simulink model "test"  (Simulink 10.1)
settings: Solver=FixedStepAuto  StartTime=0.0  StopTime=Config.simulationTime  FixedStep=Config.tStep  RelTol=1e-3
InitFcn:
  | init
undefined symbols (not defined in the file or in its folder): Config, confVisualizer, DiscIntNeverNeededParam
libraries: WBToolboxLibrary x12
settings Model: Creator=giuseppe  LastModifiedBy=giuseppe
settings DataIOCC: SaveFormat=Dataset  ReturnWorkspaceOutputs=on
settings OptimizationCC: LifeSpan=auto
settings DebuggingCC: UnderspecifiedInitializationDetection=Simplified  MergeDetectMultiDrivingBlocksExec=error  SFUnexpectedBacktrackingDiag=error  SFNoUnconditionalDefaultTransitionDiag=error  SFExecutionAtInitializationDiag=warning  ArithmeticOperatorsInVariantConditions=error
settings HardwareCC: ProdBitPerPointer=64  ProdBitPerSizeT=64  ProdBitPerPtrDiffT=64  ProdLargestAtomicFloat=Float  ProdIntDivRoundTo=Zero  ProdEndianess=LittleEndian  ProdWordSize=64  ProdHWDeviceType=Intel->x86-64 (Windows64)
settings ModelReferenceCC: PropagateSignalLabelsOutOfModel=on
settings SFSimCC: SimUseLocalCustomCode=on  CustomCodeUndefinedFunction=FilterOut
settings RTWCC: RTWUseLocalCustomCode=on
settings CodeAppCC: StateflowObjectComments=off
settings GRTTargetCC: TargetLangStandard=C99 (ISO)  CombineOutputUpdateFcns=on  GRTInterface=off
settings ConfigComp: CovMetricSettings=dwe  CovHtmlReporting=off  CovSaveCumulativeToWorkspaceVar=off  CovSaveSingleToWorkspaceVar=off  CovExternalEMLEnable=on

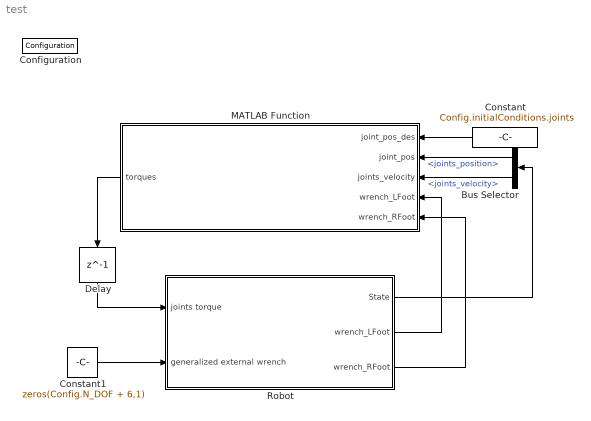
== system test ==
  Bus Selector : BusSelector  OutputSignals=joints_position,joints_velocity
  Configuration : WBToolboxLibrary/Utilities/Configuration  ConfigSource=Workspace  ConfigObject='WBTConfigRobot'
      settings: SourceProductName=WholeBodyToolbox
  Constant : Constant  Value=Config.initialConditions.joints
  Constant1 : Constant  Value=zeros(Config.N_DOF + 6,1)
  Delay : Delay  DelayLength=1  InitialCondition=zeros(23,1)
  MATLAB Function : MATLAB Function  TreatAsAtomicUnit=on
  Robot : Subsystem
  wires:
  Constant1/1 -> Robot/2(generalized external wrench)
  Bus Selector/1 -> MATLAB Function/2(joint_pos)  "<joints_position>"
  Bus Selector/2 -> MATLAB Function/3(joints_velocity)  "<joints_velocity>"
  Robot/1(State) -> Bus Selector/1
  Robot/2(wrench_LFoot) -> MATLAB Function/4(wrench_LFoot)
  Robot/3(wrench_RFoot) -> MATLAB Function/5(wrench_RFoot)
  Constant/1 -> MATLAB Function/1(joint_pos_des)
  MATLAB Function/1(torques) -> Delay/1
  Delay/1 -> Robot/1(joints torque)

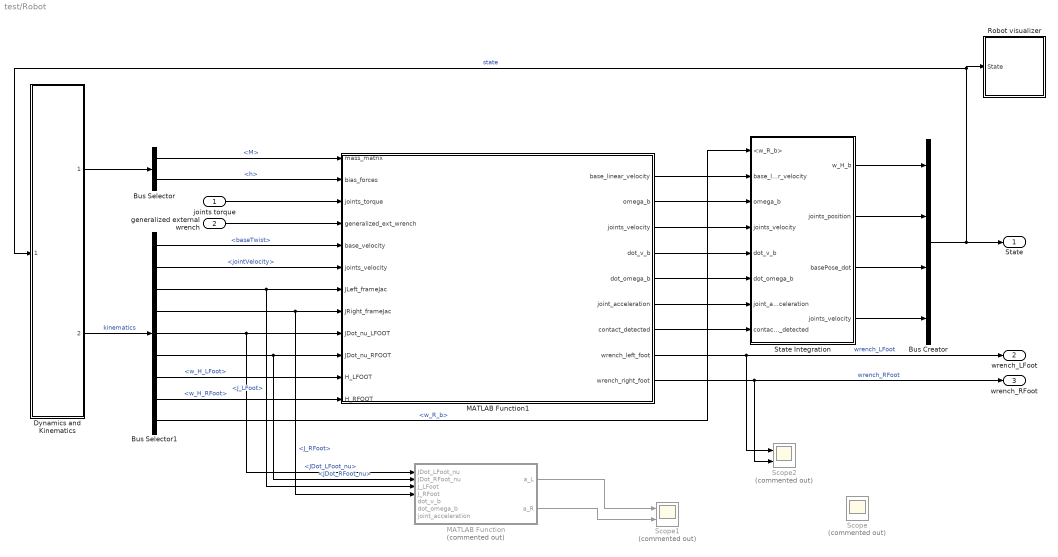
== system test/Robot ==
  joints torque : Inport
  generalized external wrench : Inport  Port=2
  Bus Creator : BusCreator  Inputs=4
  Bus Selector : BusSelector  OutputSignals=M,h
  Bus Selector1 : BusSelector  OutputSignals=baseTwist,jointVelocity,J_LFoot,J_RFoot,JDot_LFoot_nu,JDot_RFoot_nu,w_H_LFoot,w_H_RFoot,w_R_b
  Dynamics and Kinematics : Subsystem
  MATLAB Function : MATLAB Function  Commented=on  TreatAsAtomicUnit=on
  MATLAB Function1 : MATLAB Function  TreatAsAtomicUnit=on
  Robot visualizer : Subsystem  SystemSampleTime=confVisualizer.tStep
  Scope : Scope  Commented=on
  Scope1 : Scope  Commented=on  NumInputPorts=2
  Scope2 : Scope  Commented=on  NumInputPorts=2
  State Integration : Subsystem
  State : Outport
  wrench_LFoot : Outport  Port=2
  wrench_RFoot : Outport  Port=3
  wires:
  Bus Selector1/9 -> State Integration/1(<w_R_b>)  "<w_R_b>"
  State Integration/1(w_H_b) -> Bus Creator/1
  Bus Selector1/6 -> MATLAB Function/2(JDot_RFoot_nu), MATLAB Function1/10(JDot_nu_RFOOT)  "<JDot_RFoot_nu>"
  Bus Selector1/5 -> MATLAB Function/1(JDot_LFoot_nu), MATLAB Function1/9(JDot_nu_LFOOT)  "<JDot_LFoot_nu>"
  MATLAB Function1/8(wrench_left_foot) -> wrench_LFoot/1, Scope2/1  "wrench_LFoot"
  MATLAB Function1/9(wrench_right_foot) -> wrench_RFoot/1, Scope2/2  "wrench_RFoot"
  Bus Selector/1 -> MATLAB Function1/1(mass_matrix)  "<M>"
  Bus Selector/2 -> MATLAB Function1/2(bias_forces)  "<h>"
  Bus Selector1/4 -> MATLAB Function/4(J_RFoot), MATLAB Function1/8(JRight_frameJac)  "<J_RFoot>"
  Bus Creator/1 -> Robot visualizer/1(State), Dynamics and Kinematics/1(systemState), State/1  "state"
  State Integration/4("joints_velocity ") -> Bus Creator/4
  State Integration/2(joints_position) -> Bus Creator/2
  Bus Selector1/2 -> MATLAB Function1/6("joints_velocity ")  "<jointVelocity>"
  State Integration/3(basePose_dot) -> Bus Creator/3
  Bus Selector1/8 -> MATLAB Function1/12(H_RFOOT)  "<w_H_RFoot>"
  Dynamics and Kinematics/2(kinematics) -> Bus Selector1/1  "kinematics"
  generalized external wrench/1 -> MATLAB Function1/4(generalized_ext_wrench)
  Dynamics and Kinematics/1(dynamics) -> Bus Selector/1
  Bus Selector1/7 -> MATLAB Function1/11(H_LFOOT)  "<w_H_LFoot>"
  Bus Selector1/3 -> MATLAB Function/3(J_LFoot), MATLAB Function1/7(JLeft_frameJac)  "<J_LFoot>"
  Bus Selector1/1 -> MATLAB Function1/5(base_velocity)  "<baseTwist>"
  joints torque/1 -> MATLAB Function1/3(joints_torque)
  MATLAB Function/1(a_L) -> Scope1/1
  MATLAB Function/2(a_R) -> Scope1/2
  MATLAB Function1/7(contact_detected) -> State Integration/8(contact_detected)
  MATLAB Function1/1(base_linear_velocity) -> State Integration/2(base_linear_velocity)
  MATLAB Function1/2(omega_b) -> State Integration/3(omega_b)
  MATLAB Function1/3(joints_velocity) -> State Integration/4(joints_velocity)
  MATLAB Function1/4(dot_v_b) -> State Integration/5(dot_v_b)
  MATLAB Function1/5(dot_omega_b) -> State Integration/6(dot_omega_b)
  MATLAB Function1/6(joint_acceleration) -> State Integration/7(joint_acceleration)

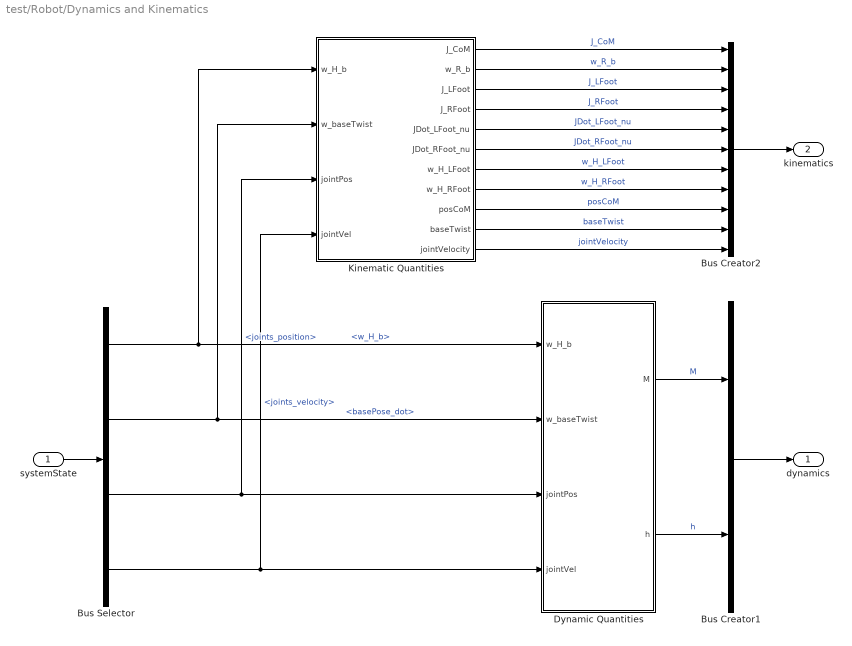
== system test/Robot/Dynamics and Kinematics ==
  systemState : Inport
  Bus Creator1 : BusCreator  Inputs=2
  Bus Creator2 : BusCreator  Inputs=11
  Bus Selector : BusSelector  OutputSignals=w_H_b,basePose_dot,joints_position,joints_velocity
  Dynamic Quantities : Subsystem
  Kinematic Quantities : Subsystem
  dynamics : Outport  VectorParamsAs1DForOutWhenUnconnected=off
  kinematics : Outport  Port=2  VectorParamsAs1DForOutWhenUnconnected=off
  wires:
  systemState/1 -> Bus Selector/1
  Bus Selector/1 -> Dynamic Quantities/1(w_H_b), Kinematic Quantities/1(w_H_b)  "<w_H_b>"
  Bus Selector/3 -> Dynamic Quantities/3(jointPos), Kinematic Quantities/3(jointPos)  "<joints_position>"
  Dynamic Quantities/2("h ") -> Bus Creator1/2  "h"
  Dynamic Quantities/1(M) -> Bus Creator1/1  "M"
  Bus Creator1/1 -> dynamics/1
  Bus Creator2/1 -> kinematics/1
  Kinematic Quantities/1(J_CoM) -> Bus Creator2/1  "J_CoM"
  Kinematic Quantities/2(w_R_b) -> Bus Creator2/2  "w_R_b"
  Kinematic Quantities/3(J_LFoot) -> Bus Creator2/3  "J_LFoot"
  Kinematic Quantities/4(J_RFoot) -> Bus Creator2/4  "J_RFoot"
  Kinematic Quantities/5(JDot_LFoot_nu) -> Bus Creator2/5  "JDot_LFoot_nu"
  Kinematic Quantities/6(JDot_RFoot_nu) -> Bus Creator2/6  "JDot_RFoot_nu"
  Kinematic Quantities/7(w_H_LFoot) -> Bus Creator2/7  "w_H_LFoot"
  Kinematic Quantities/8(w_H_RFoot) -> Bus Creator2/8  "w_H_RFoot"
  Kinematic Quantities/9(posCoM) -> Bus Creator2/9  "posCoM"
  Bus Selector/2 -> Kinematic Quantities/2(w_baseTwist), Dynamic Quantities/2(w_baseTwist)  "<basePose_dot>"
  Bus Selector/4 -> Kinematic Quantities/4(jointVel), Dynamic Quantities/4(jointVel)  "<joints_velocity>"
  Kinematic Quantities/10(baseTwist) -> Bus Creator2/10  "baseTwist"
  Kinematic Quantities/11(jointVelocity) -> Bus Creator2/11  "jointVelocity"

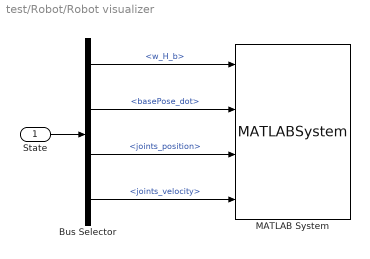
== system test/Robot/Robot visualizer ==
  State : Inport
  Bus Selector : BusSelector  OutputSignals=w_H_b,basePose_dot,joints_position,joints_velocity
  MATLAB System : MATLABSystem  System=Visualizer  config=confVisualizer  SimulateUsing=Interpreted execution
      mask Type: Visualizer
      mask Display:
      | disp(['Robot' char(10) 'Visualizer']);
      | port_label('input',1,'world_H_base');
      | port_label('input',2,'base_velocity');
      | port_label('input',3,'joints_positions');
      | port_label('input',4,'joints_velocity');
  wires:
  State/1 -> Bus Selector/1
  Bus Selector/1 -> MATLAB System/1  "<w_H_b>"
  Bus Selector/3 -> MATLAB System/3  "<joints_position>"
  Bus Selector/2 -> MATLAB System/2  "<basePose_dot>"
  Bus Selector/4 -> MATLAB System/4  "<joints_velocity>"

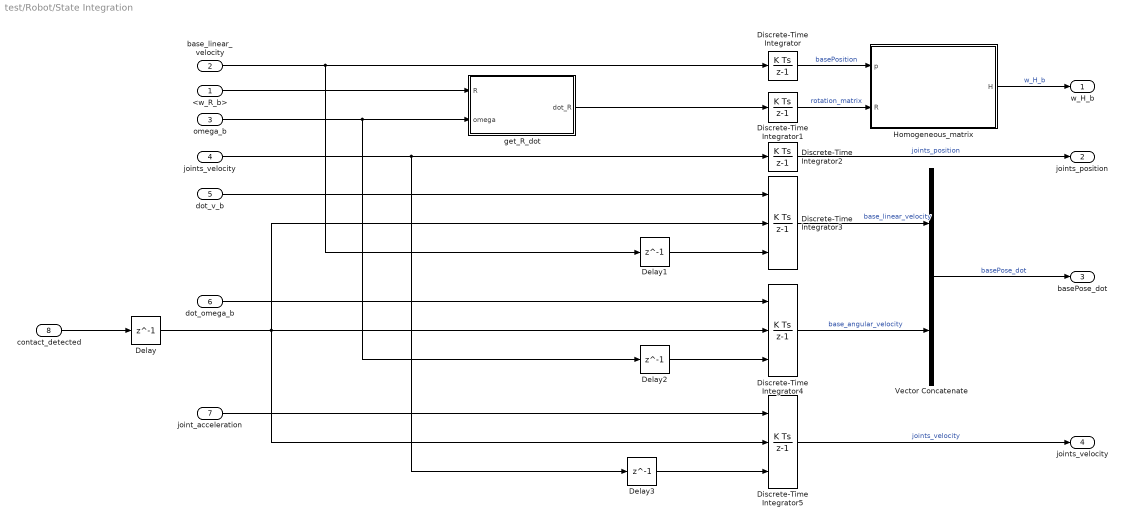
== system test/Robot/State Integration ==
  <w_R_b> : Inport
  base_linear_velocity : Inport  Port=2
  omega_b : Inport  Port=3
  joints_velocity : Inport  Port=4
  dot_v_b : Inport  Port=5
  dot_omega_b : Inport  Port=6
  joint_acceleration : Inport  Port=7
  contact_detected : Inport  Port=8
  Delay : Delay  DelayLength=1  InitialCondition=0
  Delay1 : Delay  DelayLength=1  InitialCondition=Config.initialConditions.base_linear_velocity
  Delay2 : Delay  DelayLength=1  InitialCondition=Config.initialConditions.base_angular_velocity
  Delay3 : Delay  DelayLength=1  InitialCondition=Config.initialConditions.joints_velocity
  Discrete-Time Integrator : DiscreteIntegrator  InitialCondition=Config.initialConditions.base_position  SampleTime=-1  ICPrevOutput=DiscIntNeverNeededParam  ICPrevScaledInput=DiscIntNeverNeededParam
  Discrete-Time Integrator1 : DiscreteIntegrator  InitialCondition=Config.initialConditions.orientation  SampleTime=-1  ICPrevOutput=DiscIntNeverNeededParam  ICPrevScaledInput=DiscIntNeverNeededParam
  Discrete-Time Integrator2 : DiscreteIntegrator  InitialCondition=Config.initialConditions.joints  SampleTime=-1  ICPrevOutput=DiscIntNeverNeededParam  ICPrevScaledInput=DiscIntNeverNeededParam
  Discrete-Time Integrator3 : DiscreteIntegrator  ExternalReset=rising  InitialConditionSource=external  InitialCondition=Config.initialConditions.base_linear_velocity  SampleTime=-1  ICPrevOutput=DiscIntNeverNeededParam  ICPrevScaledInput=DiscIntNeverNeededParam
  Discrete-Time Integrator4 : DiscreteIntegrator  ExternalReset=rising  InitialConditionSource=external  InitialCondition=Config.initialConditions.base_angular_velocity  SampleTime=-1  ICPrevOutput=DiscIntNeverNeededParam  ICPrevScaledInput=DiscIntNeverNeededParam
  Discrete-Time Integrator5 : DiscreteIntegrator  ExternalReset=rising  InitialConditionSource=external  InitialCondition=Config.initialConditions.joints_velocity  SampleTime=-1  ICPrevOutput=DiscIntNeverNeededParam  ICPrevScaledInput=DiscIntNeverNeededParam
  "Homogeneous_matrix " : MATLAB Function  TreatAsAtomicUnit=on
  Vector Concatenate : Concatenate
  "get_R_dot " : MATLAB Function  TreatAsAtomicUnit=on
  w_H_b : Outport  VectorParamsAs1DForOutWhenUnconnected=off
  joints_position : Outport  Port=2  VectorParamsAs1DForOutWhenUnconnected=off
  basePose_dot : Outport  Port=3  VectorParamsAs1DForOutWhenUnconnected=off
  "joints_velocity " : Outport  Port=4  VectorParamsAs1DForOutWhenUnconnected=off
  wires:
  Discrete-Time Integrator3/1 -> Vector Concatenate/1  "base_linear_velocity"
  omega_b/1 -> "get_R_dot "/2(omega), Delay2/1
  Discrete-Time Integrator5/1 -> "joints_velocity "/1  "joints_velocity"
  dot_v_b/1 -> Discrete-Time Integrator3/1
  Discrete-Time Integrator2/1 -> joints_position/1  "joints_position"
  <w_R_b>/1 -> "get_R_dot "/1(R)
  Discrete-Time Integrator4/1 -> Vector Concatenate/2  "base_angular_velocity"
  "Homogeneous_matrix "/1(H) -> w_H_b/1  "w_H_b"
  Vector Concatenate/1 -> basePose_dot/1  "basePose_dot"
  joints_velocity/1 -> Discrete-Time Integrator2/1, Delay3/1
  Discrete-Time Integrator/1 -> "Homogeneous_matrix "/1(p)  "basePosition"
  "get_R_dot "/1(dot_R) -> Discrete-Time Integrator1/1
  dot_omega_b/1 -> Discrete-Time Integrator4/1
  joint_acceleration/1 -> Discrete-Time Integrator5/1
  Discrete-Time Integrator1/1 -> "Homogeneous_matrix "/2(R)  "rotation_matrix"
  base_linear_velocity/1 -> Discrete-Time Integrator/1, Delay1/1
  contact_detected/1 -> Delay/1
  Delay/1 -> Discrete-Time Integrator3/2, Discrete-Time Integrator4/2, Discrete-Time Integrator5/2
  Delay1/1 -> Discrete-Time Integrator3/3
  Delay2/1 -> Discrete-Time Integrator4/3
  Delay3/1 -> Discrete-Time Integrator5/3

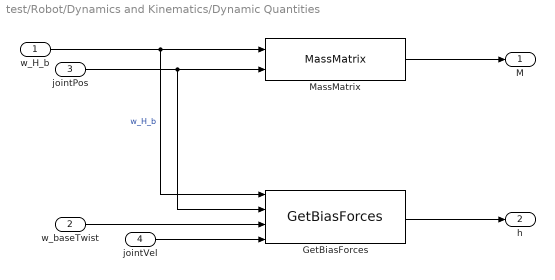
== system test/Robot/Dynamics and Kinematics/Dynamic Quantities ==
  w_H_b : Inport
  w_baseTwist : Inport  Port=2
  jointPos : Inport  Port=3
  jointVel : Inport  Port=4
  GetBiasForces : WBToolboxLibrary/Model/Dynamics/GetBiasForces
      settings: SourceProductName=WholeBodyToolbox
  MassMatrix : WBToolboxLibrary/Model/Dynamics/MassMatrix
      settings: SourceProductName=WholeBodyToolbox
  M : Outport  VectorParamsAs1DForOutWhenUnconnected=off
  "h " : Outport  Port=2  VectorParamsAs1DForOutWhenUnconnected=off
  wires:
  w_H_b/1 -> GetBiasForces/1, MassMatrix/1  "w_H_b"
  w_baseTwist/1 -> GetBiasForces/3
  jointVel/1 -> GetBiasForces/4
  MassMatrix/1 -> M/1
  GetBiasForces/1 -> "h "/1
  jointPos/1 -> GetBiasForces/2, MassMatrix/2

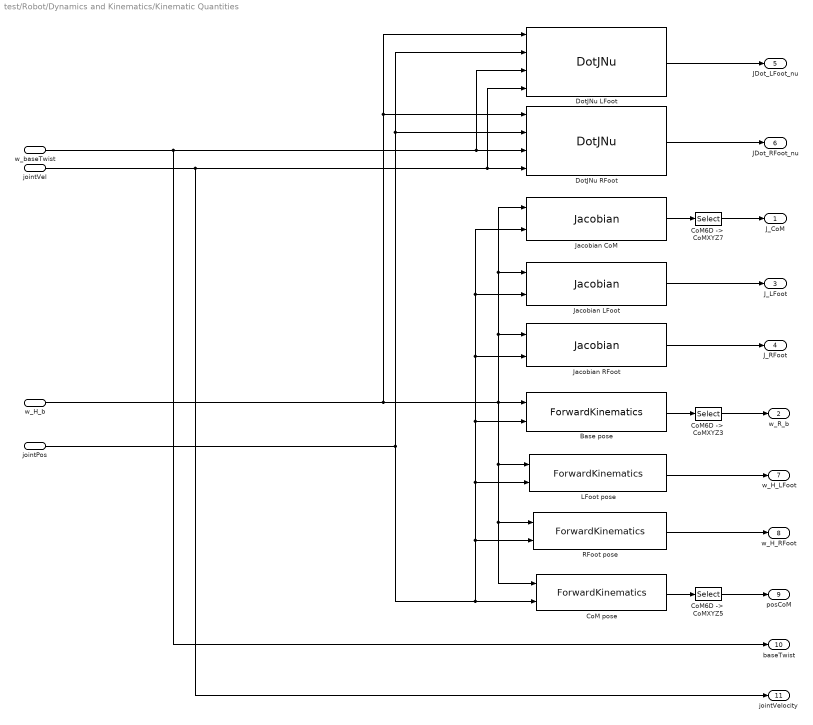
== system test/Robot/Dynamics and Kinematics/Kinematic Quantities ==
  w_H_b : Inport
  w_baseTwist : Inport  Port=2
  jointPos : Inport  Port=3
  jointVel : Inport  Port=4
  Base pose : WBToolboxLibrary/Model/Kinematics/ForwardKinematics  frameName=Frames.BASE_LINK
      settings: SourceProductName=WholeBodyToolbox
  CoM pose : WBToolboxLibrary/Model/Kinematics/ForwardKinematics  frameName=Frames.COM_FRAME
      settings: SourceProductName=WholeBodyToolbox
  "CoM6D ->  CoMXYZ3" : Selector  NumberOfDimensions=2  InputPortWidth=7  IndexOptions=Index vector (dialog),Index vector (dialog)  Indices=[1 2 3],[1 2 3]  OutputSizes=1,1
  "CoM6D ->  CoMXYZ5" : Selector  NumberOfDimensions=2  InputPortWidth=7  IndexOptions=Index vector (dialog),Index vector (dialog)  Indices=[1 2 3],[4]  OutputSizes=1,1
  "CoM6D ->  CoMXYZ7" : Selector  NumberOfDimensions=2  InputPortWidth=7  IndexOptions=Index vector (dialog),Index vector (dialog)  Indices=[1 2 3],[1:6+Config.N_DOF]  OutputSizes=1,1
  DotJNu LFoot : WBToolboxLibrary/Model/Jacobians/DotJNu  frameName=Frames.LFOOT_FRAME
      settings: SourceProductName=WholeBodyToolbox
  DotJNu RFoot : WBToolboxLibrary/Model/Jacobians/DotJNu  frameName=Frames.RFOOT_FRAME
      settings: SourceProductName=WholeBodyToolbox
  Jacobian CoM : WBToolboxLibrary/Model/Jacobians/Jacobian  frameName=Frames.COM_FRAME
      settings: SourceProductName=WholeBodyToolbox
  Jacobian LFoot : WBToolboxLibrary/Model/Jacobians/Jacobian  frameName=Frames.LFOOT_FRAME
      settings: SourceProductName=WholeBodyToolbox
  Jacobian RFoot : WBToolboxLibrary/Model/Jacobians/Jacobian  frameName=Frames.RFOOT_FRAME
      settings: SourceProductName=WholeBodyToolbox
  LFoot pose : WBToolboxLibrary/Model/Kinematics/ForwardKinematics  frameName=Frames.LFOOT_FRAME
      settings: SourceProductName=WholeBodyToolbox
  RFoot pose : WBToolboxLibrary/Model/Kinematics/ForwardKinematics  frameName=Frames.RFOOT_FRAME
      settings: SourceProductName=WholeBodyToolbox
  J_CoM : Outport  VectorParamsAs1DForOutWhenUnconnected=off
  w_R_b : Outport  Port=2  VectorParamsAs1DForOutWhenUnconnected=off
  J_LFoot : Outport  Port=3  VectorParamsAs1DForOutWhenUnconnected=off
  J_RFoot : Outport  Port=4  VectorParamsAs1DForOutWhenUnconnected=off
  JDot_LFoot_nu : Outport  Port=5  VectorParamsAs1DForOutWhenUnconnected=off
  JDot_RFoot_nu : Outport  Port=6  VectorParamsAs1DForOutWhenUnconnected=off
  w_H_LFoot : Outport  Port=7  VectorParamsAs1DForOutWhenUnconnected=off
  w_H_RFoot : Outport  Port=8  VectorParamsAs1DForOutWhenUnconnected=off
  posCoM : Outport  Port=9  VectorParamsAs1DForOutWhenUnconnected=off
  baseTwist : Outport  Port=10
  jointVelocity : Outport  Port=11
  wires:
  CoM pose/1 -> "CoM6D ->  CoMXYZ5"/1
  "CoM6D ->  CoMXYZ5"/1 -> posCoM/1
  w_H_b/1 -> DotJNu LFoot/1, DotJNu RFoot/1, Jacobian LFoot/1, Jacobian CoM/1, Jacobian RFoot/1, CoM pose/1, RFoot pose/1, LFoot pose/1, Base pose/1
  "CoM6D ->  CoMXYZ3"/1 -> w_R_b/1
  jointPos/1 -> LFoot pose/2, Jacobian RFoot/2, Jacobian LFoot/2, Jacobian CoM/2, Base pose/2, RFoot pose/2, CoM pose/2, DotJNu RFoot/2, DotJNu LFoot/2
  Jacobian CoM/1 -> "CoM6D ->  CoMXYZ7"/1
  Jacobian RFoot/1 -> J_RFoot/1
  Jacobian LFoot/1 -> J_LFoot/1
  DotJNu RFoot/1 -> JDot_RFoot_nu/1
  DotJNu LFoot/1 -> JDot_LFoot_nu/1
  jointVel/1 -> jointVelocity/1, DotJNu RFoot/4, DotJNu LFoot/4
  w_baseTwist/1 -> baseTwist/1, DotJNu LFoot/3, DotJNu RFoot/3
  RFoot pose/1 -> w_H_RFoot/1
  LFoot pose/1 -> w_H_LFoot/1
  Base pose/1 -> "CoM6D ->  CoMXYZ3"/1
  "CoM6D ->  CoMXYZ7"/1 -> J_CoM/1

== matlab function Robot/MATLAB Function1 ==
  data: base_linear_velocity output double; mass_matrix input double; bias_forces input double; joints_torque input double; generalized_ext_wrench input double; base_velocity input double; joints_velocity input double; JLeft_frameJac input double; JRight_frameJac input double; JDot_nu_LFOOT input double; JDot_nu_RFOOT input double; H_LFOOT input double; H_RFOOT input double; Config parameter double; omega_b output double; joints_velocity output double; dot_v_b output double; dot_omega_b output double; joint_acceleration output double; contact_detected output double; wrench_left_foot output double; wrench_right_foot output double
function [base_linear_velocity, omega_b, joints_velocity, dot_v_b, dot_omega_b, joint_acceleration, ...
    contact_detected, wrench_left_foot, wrench_right_foot] = ...
    forward_and_contact_dynamics(mass_matrix, bias_forces, joints_torque, generalized_ext_wrench, ...
    base_velocity, joints_velocity, JLeft_frameJac, JRight_frameJac, JDot_nu_LFOOT, JDot_nu_RFOOT, H_LFOOT, H_RFOOT, Config)

[base_linear_velocity, omega_b, joints_velocity, dot_v_b, dot_omega_b, joint_acceleration, ...
    contact_detected, wrench_left_foot, wrench_right_foot] = ...
    forward_and_contact_dynamics(mass_matrix, bias_forces, joints_torque, generalized_ext_wrench, ...
    base_velocity, joints_velocity, JLeft_frameJac, JRight_frameJac, JDot_nu_LFOOT, JDot_nu_RFOOT, H_LFOOT, H_RFOOT, Config);
end

== matlab function Robot/MATLAB Function ==
  data: JDot_LFoot_nu input double; a_L output double; JDot_RFoot_nu input double; J_LFoot input double; J_RFoot input double; dot_v_b input double; dot_omega_b input double; joint_acceleration input double; a_R output double
function [a_L, a_R] = fcn(JDot_LFoot_nu, JDot_RFoot_nu, J_LFoot, J_RFoot, dot_v_b, dot_omega_b, joint_acceleration)
a_L = JDot_LFoot_nu + J_LFoot*[dot_v_b; dot_omega_b; joint_acceleration];

a_R = JDot_RFoot_nu + J_RFoot*[dot_v_b; dot_omega_b; joint_acceleration];

== matlab function MATLAB Function ==
  data: torques output double; joint_pos_des input double; joint_pos input double; joints_velocity input double; wrench_LFoot input double; wrench_RFoot input double
function torques = dummy_torque_control(joint_pos_des, joint_pos, joints_velocity, wrench_LFoot, wrench_RFoot)

joints_pos_error = (joint_pos_des - joint_pos); 
% 
% J = [Jl; Jr];
% 
KP = 1;
KD = 2*sqrt(KP);
% 
% acceleration_star = KP*(joints_pos_error) - KD*joints_velocity;
% 
% S = [zeros(6,23); eye(23)];

torques = KP*(joints_pos_error) - KD*joints_velocity;

== matlab function Robot/State Integration/get_R_dot  ==
  data: R input double size=[3, 3]; omega input double size=[3, 1]; dot_R output double size=[3, 3]
function dot_R = get_R_dot(R, omega)
    dot_R = get_R_dot(R, omega);
end

== matlab function Robot/State Integration/Homogeneous_matrix  ==
  data: p input double; H output double; R input double
function H = Rp2Hom(p, R)
    H = Rp2Hom(p, R);
end
